simulink subsystem "Line_Following_Drone_Model"  (R2019b)
settings: Solver=VariableStepAuto  StartTime=0.0  StopTime=10.0  RelTol=1e-3
values from neighbouring files (symbols this model uses):
  Kd = 2    [shared_variables.m]
  Kp = 1    [shared_variables.m]
  pathDirection = 1.0 2.0    [Lab_5_Model_System_Data.sldd]    (also in Lab_5_Real_System_Data.sldd)
  pathReferencePoint = 0.0 0.0    [Lab_5_Model_System_Data.sldd]    (also in Lab_5_Real_System_Data.sldd)
  V = 40.0    [Lab_5_Model_System_Data.sldd]    (also in Lab_5_Real_System_Data.sldd)
  windRadial = 270.0    [Lab_5_Model_System_Data.sldd]    (also in Lab_5_Real_System_Data.sldd)
  windSpeed = 15.0    [Lab_5_Model_System_Data.sldd]    (also in Lab_5_Real_System_Data.sldd)
  x0 = 0.0 0.0 1.1071487177940904    [Lab_5_Model_System_Data.sldd]    (also in Lab_5_Real_System_Data.sldd = 1.0 0.0 0.78539816339744828)
libraries: dspmathops x3
settings Model: Creator=rolle  LastModifiedBy=rollends

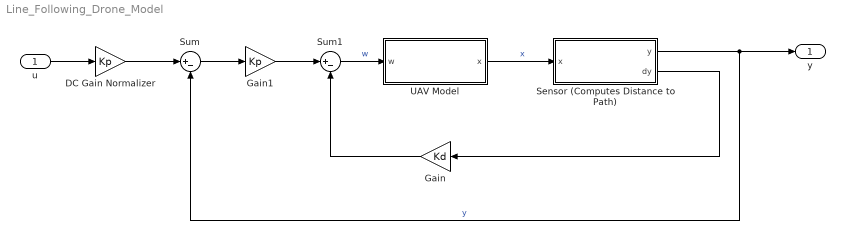
== system Line_Following_Drone_Model ==
  u : Inport
  DC Gain Normalizer : Gain  Gain=Kp
  Gain : Gain  Gain=Kd
  Gain1 : Gain  Gain=Kp
  Sensor (Computes Distance to Path) : Subsystem
  Sum : Sum  Inputs=|+-
  Sum1 : Sum  Inputs=|+-
  UAV Model : Subsystem
  y : Outport
  wires:
  UAV Model/1(x) -> Sensor (Computes Distance to Path)/1(x)  "x"
  Sensor (Computes Distance to Path)/1(y) -> Sum/2, y/1  "y"
  Sum1/1 -> UAV Model/1(w)  "w"
  Sum/1 -> Gain1/1
  u/1 -> DC Gain Normalizer/1
  Sensor (Computes Distance to Path)/2(dy) -> Gain/1
  Gain/1 -> Sum1/2
  Gain1/1 -> Sum1/1
  DC Gain Normalizer/1 -> Sum/1

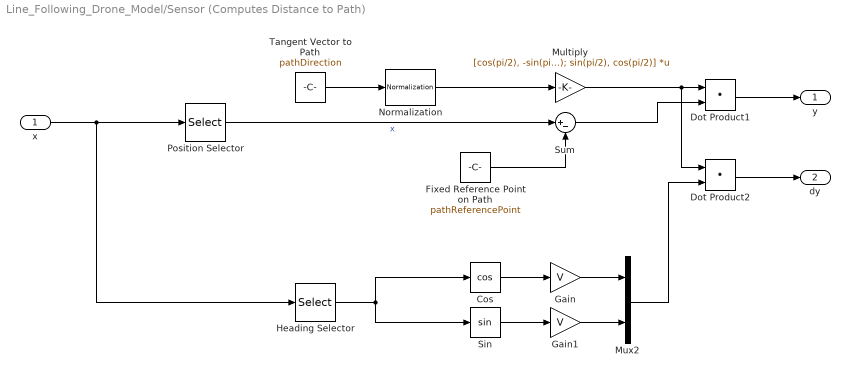
== system Line_Following_Drone_Model/Sensor (Computes Distance to Path) ==
  x : Inport
  Cos : Trigonometry  Operator=cos
  Dot Product1 : DotProduct  InputSameDT=on  OutDataTypeStr=Inherit: Inherit via internal rule
  Dot Product2 : DotProduct  InputSameDT=on  OutDataTypeStr=Inherit: Inherit via internal rule
  Fixed Reference Point on Path : Constant  Value=pathReferencePoint
  Gain : Gain  Gain=V
  Gain1 : Gain  Gain=V
  Heading Selector : Selector  InputPortWidth=3  IndexOptions=Index vector (dialog)  Indices=3  OutputSizes=1
  Multiply : Gain  Gain=[cos(pi/2), -sin(pi/2); sin(pi/2), cos(pi/2)]  Multiplication=Matrix(K*u)
  Mux2 : Mux  Inputs=2
  Normalization : dspmathops/Normalization  NormType=2-norm  Bias=1e-10  NormOver=Each column  Dimension=1  roundingMode=Floor  overflowMode=off  accumDataTypeStr=Inherit: Same as product output  accumLastDataTypeStr=Inherit: Same as product output  outputDataTypeStr=Inherit: Same as product output  outputMin=[]  outputMax=[]  outputLastDataTypeStr=Inherit: Same as product output
  Position Selector : Selector  InputPortWidth=3  IndexOptions=Index vector (dialog)  Indices=[1 2]  OutputSizes=1
  Sin : Trigonometry
  Sum : Sum  Inputs=|+-
  Tangent Vector to Path : Constant  Value=pathDirection
  y : Outport
  dy : Outport  Port=2
  wires:
  Dot Product2/1 -> dy/1
  Mux2/1 -> Dot Product2/2
  Sin/1 -> Gain1/1
  Cos/1 -> Gain/1
  Gain/1 -> Mux2/1
  Gain1/1 -> Mux2/2
  Heading Selector/1 -> Cos/1, Sin/1
  Position Selector/1 -> Sum/1  "x"
  Multiply/1 -> Dot Product1/1, Dot Product2/1
  Dot Product1/1 -> y/1
  Normalization/1 -> Multiply/1
  Fixed Reference Point on Path/1 -> Sum/2
  Sum/1 -> Dot Product1/2
  x/1 -> Position Selector/1, Heading Selector/1
  Tangent Vector to Path/1 -> Normalization/1

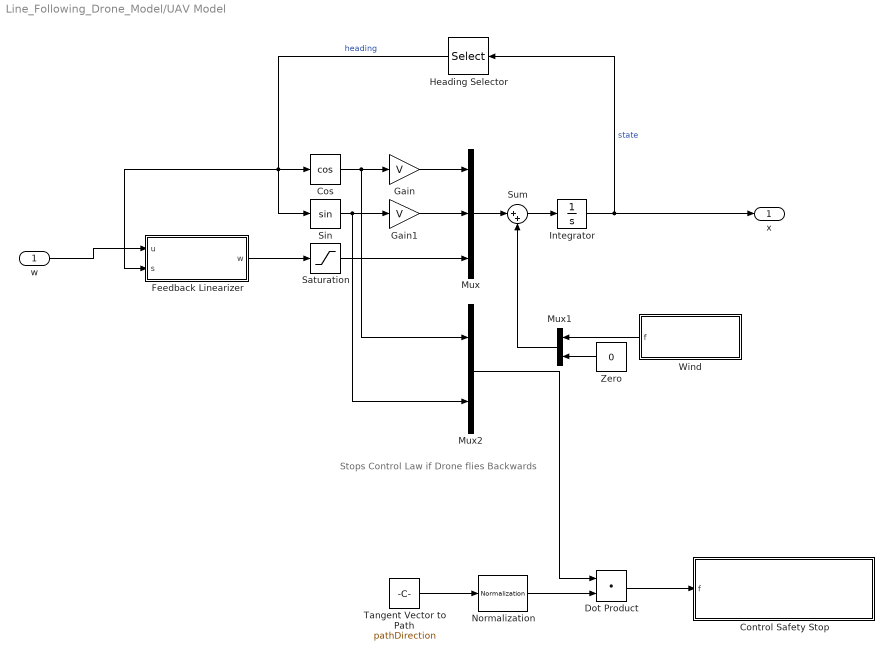
== system Line_Following_Drone_Model/UAV Model ==
  note: Stops Control Law if Drone flies Backwards
  w : Inport
  Control Safety Stop : Subsystem
  Cos : Trigonometry  Operator=cos
  Dot Product : DotProduct  InputSameDT=on  OutDataTypeStr=Inherit: Inherit via internal rule
  Feedback Linearizer : Subsystem
  Gain : Gain  Gain=V
  Gain1 : Gain  Gain=V
  Heading Selector : Selector  InputPortWidth=3  IndexOptions=Index vector (dialog)  Indices=3  OutputSizes=1
  Integrator : Integrator  InitialCondition=x0
  Mux : Mux  Inputs=3
  Mux1 : Mux  Inputs=2
  Mux2 : Mux  Inputs=2
  Normalization : dspmathops/Normalization  NormType=2-norm  Bias=1e-10  NormOver=Each column  Dimension=1  roundingMode=Floor  overflowMode=off  accumDataTypeStr=Inherit: Same as product output  accumLastDataTypeStr=Inherit: Same as product output  outputDataTypeStr=Inherit: Same as product output  outputMin=[]  outputMax=[]  outputLastDataTypeStr=Inherit: Same as product output
  Saturation : Saturate  UpperLimit=pi  LowerLimit=-pi
  Sin : Trigonometry
  Sum : Sum  Inputs=|++
  Tangent Vector to Path : Constant  Value=pathDirection
  Wind : Subsystem
  Zero : Constant  Value=0  OutDataTypeStr=Inherit: Inherit via back propagation
  x : Outport
  wires:
  Feedback Linearizer/1(w) -> Saturation/1
  w/1 -> Feedback Linearizer/1(u)
  Saturation/1 -> Mux/3
  Mux2/1 -> Dot Product/1
  Normalization/1 -> Dot Product/2
  Dot Product/1 -> Control Safety Stop/1(f)
  Tangent Vector to Path/1 -> Normalization/1
  Zero/1 -> Mux1/2
  Mux1/1 -> Sum/2
  Wind/1(f) -> Mux1/1
  Sum/1 -> Integrator/1
  Mux/1 -> Sum/1
  Gain1/1 -> Mux/2
  Sin/1 -> Gain1/1, Mux2/2
  Gain/1 -> Mux/1
  Cos/1 -> Gain/1, Mux2/1
  Heading Selector/1 -> Cos/1, Sin/1, Feedback Linearizer/2(s)  "heading"
  Integrator/1 -> Heading Selector/1, x/1  "state"

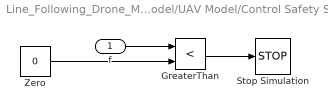
== system Line_Following_Drone_Model/UAV Model/Control Safety Stop ==
  f : Inport
  GreaterThan : RelationalOperator  Operator=<  OutDataTypeStr=boolean  RndMeth=Simplest
  Stop Simulation : Stop
  Zero : Constant  Value=0
  wires:
  Zero/1 -> GreaterThan/2
  f/1 -> GreaterThan/1
  GreaterThan/1 -> Stop Simulation/1

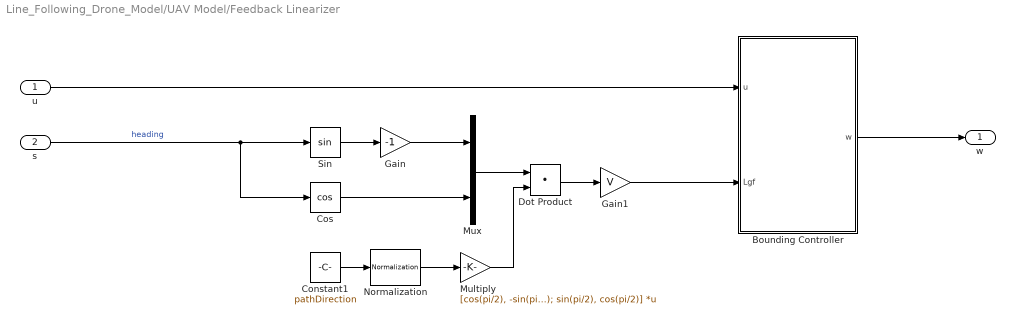
== system Line_Following_Drone_Model/UAV Model/Feedback Linearizer ==
  u : Inport
  s : Inport  Port=2
  Bounding Controller : MATLAB Function  TreatAsAtomicUnit=on
  Constant1 : Constant  Value=pathDirection
  Cos : Trigonometry  Operator=cos
  Dot Product : DotProduct  InputSameDT=on  OutDataTypeStr=Inherit: Inherit via internal rule
  Gain : Gain  Gain=-1
  Gain1 : Gain  Gain=V
  Multiply : Gain  Gain=[cos(pi/2), -sin(pi/2); sin(pi/2), cos(pi/2)]  Multiplication=Matrix(K*u)
  Mux : Mux  Inputs=2
  Normalization : dspmathops/Normalization  NormType=2-norm  Bias=1e-10  NormOver=Each column  Dimension=1  roundingMode=Floor  overflowMode=off  accumDataTypeStr=Inherit: Same as product output  accumLastDataTypeStr=Inherit: Same as product output  outputDataTypeStr=Inherit: Same as product output  outputMin=[]  outputMax=[]  outputLastDataTypeStr=Inherit: Same as product output
  Sin : Trigonometry
  w : Outport
  wires:
  Multiply/1 -> Dot Product/2
  u/1 -> Bounding Controller/1(u)
  Gain1/1 -> Bounding Controller/2(Lgf)
  Bounding Controller/1(w) -> w/1
  Dot Product/1 -> Gain1/1
  Normalization/1 -> Multiply/1
  Constant1/1 -> Normalization/1
  Mux/1 -> Dot Product/1
  Gain/1 -> Mux/1
  Cos/1 -> Mux/2
  s/1 -> Sin/1, Cos/1  "heading"
  Sin/1 -> Gain/1

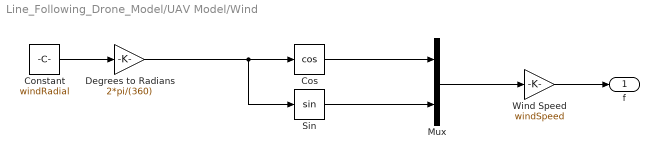
== system Line_Following_Drone_Model/UAV Model/Wind ==
  Constant : Constant  Value=windRadial
  Cos : Trigonometry  Operator=cos
  Degrees to Radians : Gain  Gain=2*pi/(360)
  Mux : Mux  Inputs=2
  Sin : Trigonometry
  Wind Speed : Gain  Gain=windSpeed
  f : Outport
  wires:
  Degrees to Radians/1 -> Cos/1, Sin/1
  Mux/1 -> Wind Speed/1
  Sin/1 -> Mux/2
  Cos/1 -> Mux/1
  Constant/1 -> Degrees to Radians/1
  Wind Speed/1 -> f/1

== matlab function Line_Following_Drone_Model/UAV Model/Feedback Linearizer/Bounding Controller ==
  data: u input; w output; Lgf input
function w = Bounding(u, Lgf)
    if abs(Lgf) <= 1e-2
        w = u / 1e-2;        
    else
        w = u / Lgf;
    end
end
